simulink model "LQG"  (R2020a)
settings: Solver=VariableStepAuto  StartTime=0.0  StopTime=5  MaxStep=0.001  RelTol=1e-3
undefined symbols (not defined in the file): A, Ao, B, Bo, C, Co, D, Do, K, Kf, x0
libraries: simulink x4
settings Model: Creator=magne  LastModifiedBy=magne

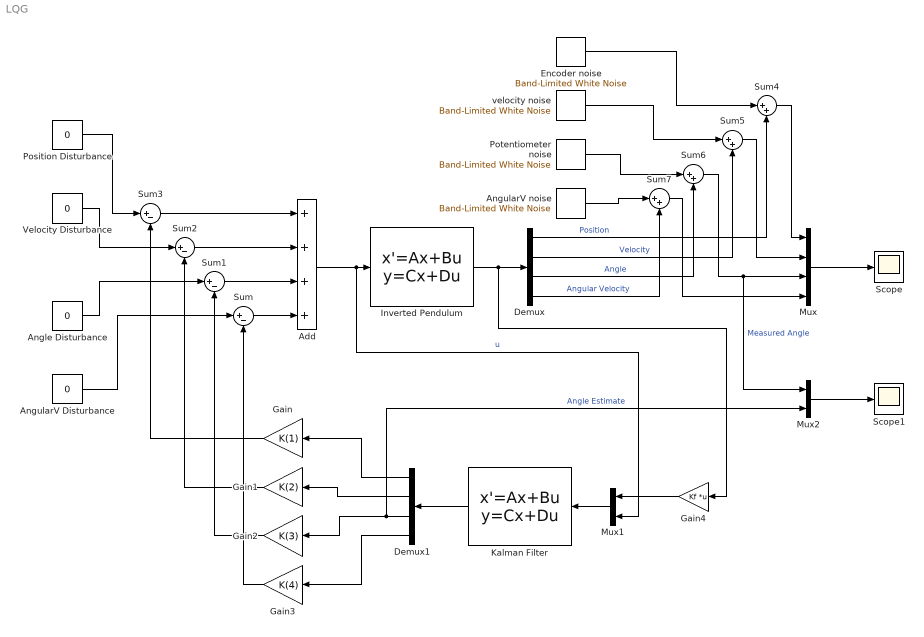
== system LQG ==
  Add : Sum  Inputs=++++
  Angle Disturbance : Constant  Value=0
  AngularV Disturbance : Constant  Value=0
  AngularV noise : simulink/Sources/Band-Limited White Noise  Cov=[0.00]  Ts=0.01  seed=[23341]
  Demux : Demux
  Demux1 : Demux
  Encoder noise : simulink/Sources/Band-Limited White Noise  Cov=[0.00]  Ts=0.01  seed=[23341]
  Gain : Gain  Gain=K(1)
  Gain1 : Gain  Gain=K(2)
  Gain2 : Gain  Gain=K(3)
  Gain3 : Gain  Gain=K(4)
  Gain4 : Gain  Gain=Kf  Multiplication=Matrix(K*u)
  Inverted Pendulum : StateSpace  A=A  B=B  C=C  D=D  InitialCondition=x0
  Kalman Filter : StateSpace  A=Ao  B=Bo  C=Co  D=Do  InitialCondition=0
  Mux : Mux
  Mux1 : Mux  Inputs=2
  Mux2 : Mux  Inputs=2
  Position Disturbance : Constant  Value=0
  Potentiometer noise : simulink/Sources/Band-Limited White Noise  Cov=[0.00]  Ts=0.01  seed=[23341]
  Scope : Scope
  Scope1 : Scope
  Sum{,1..3} (4 alike) : Sum  Inputs=|+-
  Sum{4..7} (4 alike) : Sum  Inputs=|++
  Velocity Disturbance : Constant  Value=0
  velocity noise : simulink/Sources/Band-Limited White Noise  Cov=[0.00]  Ts=0.01  seed=[23341]
  wires:
  Inverted Pendulum/1 -> Demux/1, Gain4/1
  Add/1 -> Mux1/2, Inverted Pendulum/1  "u"
  Sum/1 -> Add/4
  Sum1/1 -> Add/3
  Sum2/1 -> Add/2
  Sum3/1 -> Add/1
  AngularV Disturbance/1 -> Sum/1
  Angle Disturbance/1 -> Sum1/1
  Velocity Disturbance/1 -> Sum2/1
  Position Disturbance/1 -> Sum3/1
  Gain/1 -> Sum3/2
  Gain1/1 -> Sum2/2
  Gain2/1 -> Sum1/2
  Gain3/1 -> Sum/2
  Kalman Filter/1 -> Demux1/1
  Demux1/1 -> Gain/1
  Demux1/2 -> Gain1/1
  Demux1/3 -> Mux2/2, Gain2/1  "Angle Estimate"
  Demux1/4 -> Gain3/1
  Mux1/1 -> Kalman Filter/1
  Mux/1 -> Scope/1
  Mux2/1 -> Scope1/1
  Encoder noise/1 -> Sum4/1
  Demux/1 -> Sum4/2  "Position"
  Sum4/1 -> Mux/1
  velocity noise/1 -> Sum5/1
  Demux/2 -> Sum5/2  "Velocity"
  Sum5/1 -> Mux/2
  Potentiometer noise/1 -> Sum6/1
  Demux/3 -> Sum6/2  "Angle"
  Sum6/1 -> Mux2/1, Mux/3  "Measured Angle"
  AngularV noise/1 -> Sum7/1
  Demux/4 -> Sum7/2  "Angular Velocity"
  Sum7/1 -> Mux/4
  Gain4/1 -> Mux1/1
